simulink library "iq_splitter_4c4t_lib"  (Simulink 8.7)
settings: Solver=ode45  StartTime=0.0  StopTime=10.0  RelTol=1e-3
undefined symbols (not defined in the file): AdvDSPBChannelOutDisplay, dpoly, dspba_ChannelInVis, dspba_ChannelOutVis, dspba_internal_get_channel_ports, dspba_internal_get_demux_ports, evalAionMaskParam, latency, primtype, value
libraries: DSPBAPrim x45, Pipereg_lib x2, DSPBABase x1
settings Model: Creator=bigcat  LastModifiedBy=5g

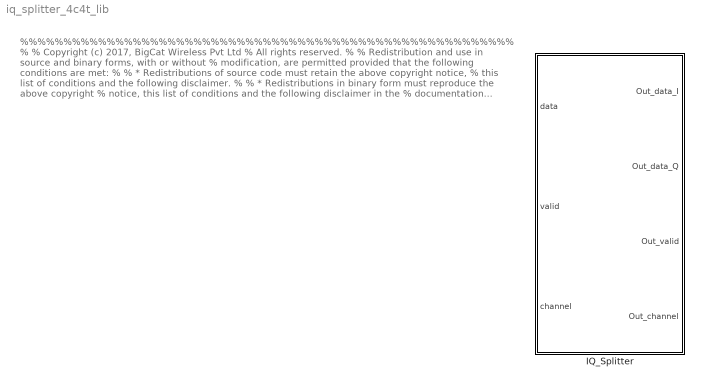
== system iq_splitter_4c4t_lib ==
  note: %%%%%%%%%%%%%%%%%%%%%%%%%%%%%%%%%%%%%%%%%%%%%%%%%%%%%%%%%
      |  %
      |  % Copyright (c) 2017, BigCat Wireless Pvt Ltd
      |  % All rights reserved.
      |  %
      |  % Redistribution and use in source and binary forms, with or without
      |  % modification, are permitted provided that the following conditions are met:
      |  %
      |  %     * Redistributions of source code must retain the above copyright notice,
      |  %       this list of conditions and the following disclaimer.
      |  %
      |  %     * Redistributions in binary form must reproduce the above copyright
      |  %       notice, this list of conditions and the following disclaimer in the
      |  %       documentation and/or other materials provided with the distribution.
      |  %
      |  %     * Neither the name of the copyright holder nor the names of its contributors
      |  %       may be used to endorse or promote products derived from this software
      |  %       without specific prior written permission.
      |  %
      |  %
      |  %
      |  % THIS SOFTWARE IS PROVIDED BY THE COPYRIGHT HOLDERS AND CONTRIBUTORS "AS IS"
      |  % AND ANY EXPRESS OR IMPLIED WARRANTIES, INCLUDING, BUT NOT LIMITED TO, THE
      |  % IMPLIED WARRANTIES OF MERCHANTABILITY AND FITNESS FOR A PARTICULAR PURPOSE ARE
      |  % DISCLAIMED. IN NO EVENT SHALL THE COPYRIGHT HOLDER OR CONTRIBUTORS BE LIABLE
      |  % FOR ANY DIRECT, INDIRECT, INCIDENTAL, SPECIAL, EXEMPLARY, OR CONSEQUENTIAL
      |  % DAMAGES (INCLUDING, BUT NOT LIMITED TO, PROCUREMENT OF SUBSTITUTE GOODS OR
      |  % SERVICES; LOSS OF USE, DATA, OR PROFITS; OR BUSINESS INTERRUPTION) HOWEVER
      |  % CAUSED AND ON ANY THEORY OF LIABILITY, WHETHER IN CONTRACT, STRICT LIABILITY,
      |  % OR TORT (INCLUDING NEGLIGENCE OR OTHERWISE) ARISING IN ANY WAY OUT OF THE USE
      |  % OF THIS SOFTWARE, EVEN IF ADVISED OF THE POSSIBILITY OF SUCH DAMAGE.
      |  %
      |   %%%%%%%%%%%%%%%%%%%%%%%%%%%%%%%%%%%%%%%%%%%%%%%%%%%%%%%%%%
  IQ_Splitter : Subsystem  mask{Latency=0, ClockMargin=0, Pipeline_stages=0}
      mask Display:
      | disp('IQ_SPLITTER');
      | port_label('input',1,'d');
      | port_label('input',2,'v');
      | port_label('input',3,'c');
      | port_label('output',1,'q_I');
      | port_label('output',2,'q_Q');
      | port_label('output',3,'q_v');
      | port_label('output',4,'q_c');

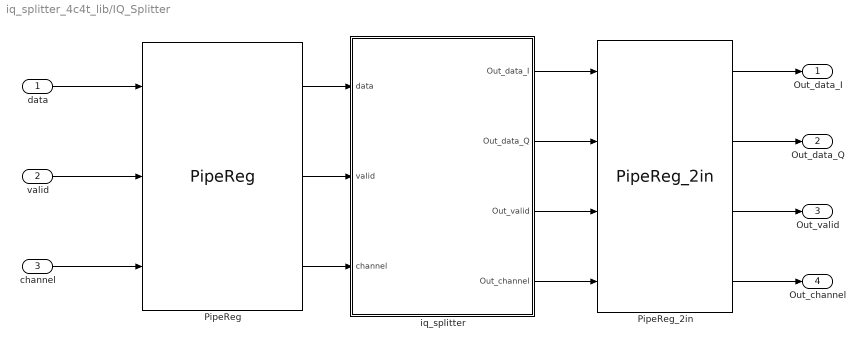
== system iq_splitter_4c4t_lib/IQ_Splitter ==
  data : Inport
  valid : Inport  Port=2
  channel : Inport  Port=3
  PipeReg : Pipereg_lib/PipeReg  NPipe=Pipeline_stages  Clock_Margin=ClockMargin
  PipeReg_2in : Pipereg_lib/PipeReg_2in  NPipe=Pipeline_stages  Clock_Margin=ClockMargin
  iq_splitter : Subsystem
  Out_data_I : Outport
  Out_data_Q : Outport  Port=2
  Out_valid : Outport  Port=3
  Out_channel : Outport  Port=4
  wires:
  PipeReg/1 -> iq_splitter/1(data)
  PipeReg/2 -> iq_splitter/2(valid)
  PipeReg/3 -> iq_splitter/3(channel)
  iq_splitter/3(Out_valid) -> PipeReg_2in/3
  iq_splitter/4(Out_channel) -> PipeReg_2in/4
  iq_splitter/1(Out_data_I) -> PipeReg_2in/1
  iq_splitter/2(Out_data_Q) -> PipeReg_2in/2
  channel/1 -> PipeReg/3
  valid/1 -> PipeReg/2
  data/1 -> PipeReg/1
  PipeReg_2in/2 -> Out_data_Q/1
  PipeReg_2in/3 -> Out_valid/1
  PipeReg_2in/4 -> Out_channel/1
  PipeReg_2in/1 -> Out_data_I/1

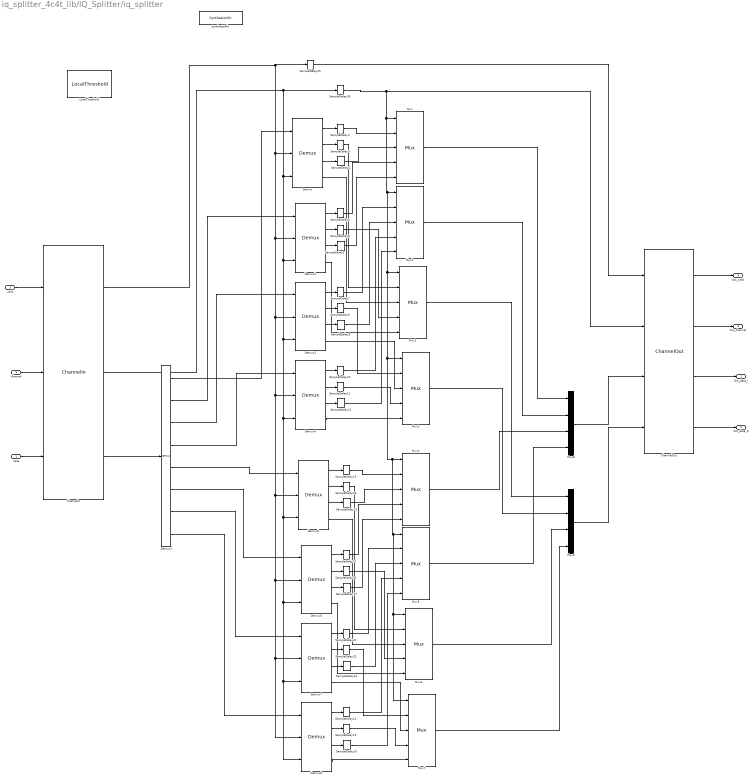
== system iq_splitter_4c4t_lib/IQ_Splitter/iq_splitter ==
  data : Inport
  valid : Inport  Port=2
  channel : Inport  Port=3
  ChannelIn : DSPBAPrim/ChannelIn  primtype=channelin  nInputs=dspba_internal_get_channel_ports(gcb)  nOutputs=dspba_internal_get_channel_ports(gcb)  omode=Inherit via internal rule  otype=sfix(16)  scale=2^-15  rndmethod=Unbiased  factor=1  satmethod=Symmetric  shift_vec=[0 1 2 -1]  value=1  inPortNames=['v'; 'c'; '0'; '1'; '2'; '3'; '4'; '5'; '6'; '7'; '8'; '9'; 'A'; 'B'; 'D'; 'E'; 'F'; 'G'; 'H'; 'I'; 'J'; 'K'; 'L'; 'M'; 'N'; 'O'; 'P'; 'Q'; 'R'; 'S'; 'T'; 'U'; 'W'; 'X'; 'Y'; 'Z']  outPortNames=['v'; 'c'; '0'; '1'; '2'; '3'; '4'; '5'; '6'; '7'; '8'; '9'; 'A'; 'B'; 'D'; 'E'; 'F'; 'G'; 'H'; 'I'; 'J'; 'K'; 'L'; 'M'; 'N'; 'O'; 'P'; 'Q'; 'R'; 'S'; 'T'; 'U'; 'W'; 'X'; 'Y'; 'Z']  dspbaimage=dspba_prim.jpg  text=fprintf('In');  style=Optimised  dataSignals=1  foldingEnabled=off  channels=1  sampleRate=200  packetBeginPresent=off  packetBeginEnabled=off  visibilities=dspba_ChannelInVis(gcb)  latencyCorrection=0  version=20141013
  ChannelOut : DSPBAPrim/ChannelOut  primtype=channelout  nInputs=dspba_internal_get_channel_ports(gcb)  nOutputs=dspba_internal_get_channel_ports(gcb)  omode=Inherit via internal rule  otype=sfix(16)  scale=2^-15  rndmethod=Unbiased  factor=1  satmethod=Symmetric  shift_vec=[0 1 2 -1]  value=2  inPortNames=['v'; 'c'; '0'; '1'; '2'; '3'; '4'; '5'; '6'; '7'; '8'; '9'; 'A'; 'B'; 'D'; 'E'; 'F'; 'G'; 'H'; 'I'; 'J'; 'K'; 'L'; 'M'; 'N'; 'O'; 'P'; 'Q'; 'R'; 'S'; 'T'; 'U'; 'W'; 'X'; 'Y'; 'Z']  outPortNames=['v'; 'c'; '0'; '1'; '2'; '3'; '4'; '5'; '6'; '7'; '8'; '9'; 'A'; 'B'; 'D'; 'E'; 'F'; 'G'; 'H'; 'I'; 'J'; 'K'; 'L'; 'M'; 'N'; 'O'; 'P'; 'Q'; 'R'; 'S'; 'T'; 'U'; 'W'; 'X'; 'Y'; 'Z']  dspbaimage=dspba_prim.jpg  text=fprintf('Out%s', AdvDSPBChannelOutDisplay(latency));  style=Optimised  dataSignals=2  foldingEnabled=off  channels=1  sampleRate=200  packetBeginPresent=off  packetBeginEnabled=off  visibilities=dspba_ChannelOutVis(gcb)  latency=21  latencyCorrection=0  version=20141013
  Demux{,1,3..8} (8 alike) : DSPBAPrim/Demux  primtype=demux  nInputs=3  nOutputs=dspba_internal_get_demux_ports(gcb)  omode=Inherit via internal rule  otype=sfix(16)  scale=2^-15  rndmethod=Unbiased  factor=1  satmethod=Symmetric  shift_vec=[0 1 2 3]  value=4  inPortNames=['q'; 'v'; 'c']  outPortNames=['c0'; 'c1']  dspbaimage=dspba_prim.jpg  text=fprintf('demux');  style=Optimised  visibilities=1536  version=20100120
  Demux2 : Demux  Outputs=8
  LocalThreshold : DSPBABase/LocalThreshold  margin=ClockMargin  delayRegOrRAMThresholdBits=10000  MediumDualMemThresholdBits=10000  LargeDualMemThresholdBits=-1  hardMultiplierThresholdLuts=-1  version=0
  Mux{,1..7} (8 alike) : DSPBAPrim/Mux  primtype=mux  nInputs=evalAionMaskParam(gcb,'value',1)+1  nOutputs=1  omode=Inherit via internal rule  otype=sfix(16)  scale=2^-15  rndmethod=Unbiased  factor=1  satmethod=Symmetric  shift_vec=[0 1 2 -1]  value=4  inPortNames=['s '; 'd0'; 'd1'; 'd2'; 'd3'; 'd4'; 'd5'; 'd6'; 'd7'; 'd8'; 'd9';]  outPortNames=[' ']  dspbaimage=dspba_prim.jpg  text=fprintf('%s', primtype);  style=Optimised  visibilities=1032  version=20131025
  Mux8 : Mux
  Mux9 : Mux
  SampleDelay{1..2,9,12..13,16..17,24} (8 alike) : DSPBAPrim/SampleDelay  primtype=sampdelay  nInputs=1  nOutputs=1  omode=Inherit via internal rule  otype=sfix(16)  scale=2^-15  rndmethod=Unbiased  factor=1  satmethod=Symmetric  shift_vec=[0 1 2 -1]  value=1  inPortNames=[' '; ' ';]  outPortNames=[' ']  dspbaimage=dspba_prim.jpg  text=dpoly(1, eye(1,value+1), 'z')  style=Optimised  visibilities=8 + 1024 + 2^17 + 2^18  flexible=off  slackgroup=0  augmented=0  version=20090407  advOptions=[]
  SampleDelay{4,6..7,10,14,19,21..22,25..26} (10 alike) : DSPBAPrim/SampleDelay  primtype=sampdelay  nInputs=1  nOutputs=1  omode=Inherit via internal rule  otype=sfix(16)  scale=2^-15  rndmethod=Unbiased  factor=1  satmethod=Symmetric  shift_vec=[0 1 2 -1]  value=3  inPortNames=[' '; ' ';]  outPortNames=[' ']  dspbaimage=dspba_prim.jpg  text=dpoly(1, eye(1,value+1), 'z')  style=Optimised  visibilities=8 + 1024 + 2^17 + 2^18  flexible=off  slackgroup=0  augmented=0  version=20090407  advOptions=[]
  SampleDelay{3,5,8,11,15,18,20,23} (8 alike) : DSPBAPrim/SampleDelay  primtype=sampdelay  nInputs=1  nOutputs=1  omode=Inherit via internal rule  otype=sfix(16)  scale=2^-15  rndmethod=Unbiased  factor=1  satmethod=Symmetric  shift_vec=[0 1 2 -1]  value=2  inPortNames=[' '; ' ';]  outPortNames=[' ']  dspbaimage=dspba_prim.jpg  text=dpoly(1, eye(1,value+1), 'z')  style=Optimised  visibilities=8 + 1024 + 2^17 + 2^18  flexible=off  slackgroup=0  augmented=0  version=20090407  advOptions=[]
  SynthesisInfo : DSPBAPrim/SynthesisInfo  primtype=synthinfo  nInputs=0  nOutputs=0  omode=Inherit via internal rule  otype=sfix(16)  scale=2^-15  rndmethod=Truncate  factor=1  satmethod=Symmetric  shift_vec=[0 1 2 -1]  value=99  inPortNames=[' '; ' ';]  outPortNames=[' ']  dspbaimage=dspba_prim_ctrl.jpg  text=fprintf('Style=%s', style);  style=Scheduled  visibilities=2^15+2^17+2^18+2^19  constraintInUse=on  constraintRelation=>  constraintLimit=Latency  bitAccurate=off  version=20090407
  Out_data_I : Outport
  Out_data_Q : Outport  Port=2
  Out_valid : Outport  Port=3
  Out_channel : Outport  Port=4
  wires:
  SampleDelay19/1 -> Mux4/2
  SampleDelay16/1 -> Mux5/5
  Demux2/7 -> Demux7/1
  Demux8/1 -> SampleDelay14/1
  Demux6/2 -> SampleDelay20/1
  Mux6/1 -> Mux9/3
  Mux5/1 -> Mux8/4
  Demux6/4 -> Mux6/5
  SampleDelay11/1 -> Mux3/4
  SampleDelay15/1 -> Mux7/4
  SampleDelay8/1 -> Mux3/2
  SampleDelay18/1 -> Mux6/2
  Demux6/3 -> SampleDelay17/1
  SampleDelay24/1 -> Mux5/3
  Mux/1 -> Mux8/1
  Demux2/6 -> Demux6/1
  SampleDelay23/1 -> Mux7/2
  SampleDelay14/1 -> Mux5/4
  valid/1 -> ChannelIn/1
  Demux/2 -> SampleDelay3/1
  ChannelOut/1 -> Out_valid/1
  Mux8/1 -> ChannelOut/3
  Demux1/4 -> Mux2/5
  SampleDelay5/1 -> Mux2/4
  SampleDelay3/1 -> Mux2/2
  SampleDelay26/1 -> ChannelOut/2, Mux4/1, Mux5/1, Mux6/1, Mux7/1, Mux3/1, Mux2/1, Mux1/1, Mux/1
  Demux/4 -> Mux2/3
  Demux4/2 -> SampleDelay11/1
  ChannelOut/2 -> Out_channel/1
  Demux2/8 -> Demux8/1
  Demux2/2 -> Demux1/1
  Demux/3 -> SampleDelay1/1
  Demux5/1 -> SampleDelay19/1
  Mux3/1 -> Mux9/2
  SampleDelay12/1 -> Mux1/5
  Demux2/5 -> Demux5/1
  Mux2/1 -> Mux9/1
  Demux1/2 -> SampleDelay5/1
  SampleDelay25/1 -> ChannelOut/1
  Demux7/4 -> Mux7/3
  ChannelOut/4 -> Out_data_Q/1
  SampleDelay6/1 -> Mux/4
  Demux3/2 -> SampleDelay8/1
  Demux7/2 -> SampleDelay23/1
  Demux3/1 -> SampleDelay7/1
  SampleDelay10/1 -> Mux1/4
  Demux3/3 -> SampleDelay9/1
  Demux7/3 -> SampleDelay24/1
  SampleDelay2/1 -> Mux/5
  Demux6/1 -> SampleDelay21/1
  Demux4/4 -> Mux3/5
  SampleDelay21/1 -> Mux4/4
  data/1 -> ChannelIn/3
  SampleDelay13/1 -> Mux4/3
  Demux/1 -> SampleDelay4/1
  Demux3/4 -> Mux3/3
  Demux8/4 -> Mux7/5
  Mux1/1 -> Mux8/2
  Demux2/3 -> Demux3/1
  SampleDelay22/1 -> Mux5/2
  Demux8/2 -> SampleDelay15/1
  channel/1 -> ChannelIn/2
  Demux4/3 -> SampleDelay12/1
  ChannelOut/3 -> Out_data_I/1
  ChannelIn/1 -> Demux/2, Demux3/2, Demux5/2, Demux6/2, Demux7/2, Demux8/2, Demux4/2, Demux1/2, SampleDelay25/1
  Demux7/1 -> SampleDelay22/1
  SampleDelay20/1 -> Mux6/4
  Demux5/4 -> Mux6/3
  ChannelIn/3 -> Demux2/1
  Demux5/2 -> SampleDelay18/1
  Demux2/1 -> Demux/1
  Demux4/1 -> SampleDelay10/1
  Demux2/4 -> Demux4/1
  SampleDelay4/1 -> Mux/2
  Mux4/1 -> Mux8/3
  Demux1/3 -> SampleDelay2/1
  SampleDelay17/1 -> Mux4/5
  SampleDelay1/1 -> Mux/3
  SampleDelay7/1 -> Mux1/2
  Demux1/1 -> SampleDelay6/1
  Demux8/3 -> SampleDelay16/1
  SampleDelay9/1 -> Mux1/3
  Demux5/3 -> SampleDelay13/1
  Mux9/1 -> ChannelOut/4
  ChannelIn/2 -> Demux/3, Demux3/3, Demux5/3, Demux6/3, Demux8/3, Demux7/3, Demux4/3, Demux1/3, SampleDelay26/1
  Mux7/1 -> Mux9/4
